simulink model "MPC_Design_1"  (R2023b)
settings: Solver=ode5  StartTime=0.0  StopTime=7  FixedStep=Ts  RelTol=1e-3
InitFcn:
  | Init_Model;
StartFcn:
  | Init_Model;
values from neighbouring files (symbols this model uses):
  ref = [0, 0]    [MPC_Design.m]
undefined symbols (not defined in the file or in its folder): Norm
libraries: slident x1, mpclib x1
settings Model: Creator=Selim  LastModifiedBy=Selim

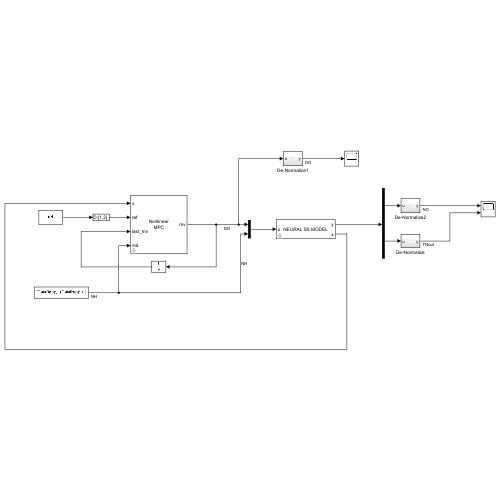
[thumbnail: Simulink's stored preview of the top-level diagram]
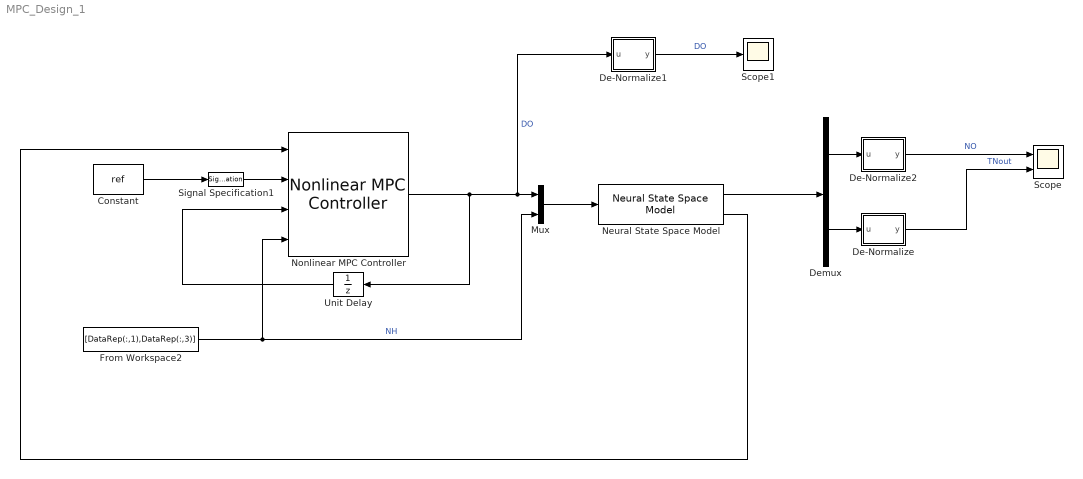
== system MPC_Design_1 ==
  Constant : Constant  Value=ref
  De-Normalize : Subsystem
  De-Normalize1 : Subsystem
  De-Normalize2 : Subsystem
  Demux : Demux  Outputs=2
  From Workspace2 : FromWorkspace  VariableName=[DataRep(:,1),DataRep(:,3)]
  Mux : Mux  Inputs=2
  Neural State Space Model : slident/Models/Neural State Space Model  sys=sys  x0type=internal  ic=x0  returnx=on  returndx=off  domain=CT  feedthroughCT=NoFT  feedthroughDT=FT
  Nonlinear MPC Controller : mpclib/Nonlinear MPC Controller  nlmpcobj=nlobj  UseObjectTs=on  UseMEX=off  md_enabled=on  mvtarget_enabled=off  param_enabled=off  cost_enabled=off  mvseq_enabled=off  stateseq_enabled=off  ovseq_enabled=off  slack_enabled=off  status_enabled=off  ov_min=off  ov_max=off  mv_min=off  mv_max=off  mvrate_min=off  mvrate_max=off  state_min=off  state_max=off  ov_weight=off  mv_weight=off  mvrate_weight=off  ecr_weight=off  nlp_initialize=off
  Scope : Scope  NumInputPorts=2
  Scope1 : Scope
  Signal Specification1 : SignalSpecification  Dimensions=[1,2]
  Unit Delay : UnitDelay  SampleTime=-1  HasFrameUpgradeWarning=on
  wires:
  Nonlinear MPC Controller/1 -> Unit Delay/1, De-Normalize1/1(u), Mux/1  "DO"
  Unit Delay/1 -> Nonlinear MPC Controller/3
  Mux/1 -> Neural State Space Model/1
  From Workspace2/1 -> Nonlinear MPC Controller/4, Mux/2  "NH"
  Demux/1 -> De-Normalize2/1(u)
  Demux/2 -> De-Normalize/1(u)
  De-Normalize2/1(y) -> Scope/1  "NO"
  De-Normalize/1(y) -> Scope/2  "TNout"
  Neural State Space Model/1 -> Demux/1
  Constant/1 -> Signal Specification1/1
  Neural State Space Model/2 -> Nonlinear MPC Controller/1
  De-Normalize1/1(y) -> Scope1/1  "DO"
  Signal Specification1/1 -> Nonlinear MPC Controller/2

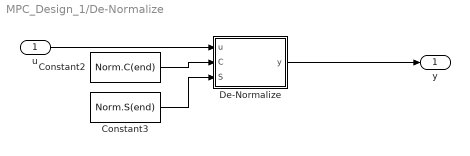
== system MPC_Design_1/De-Normalize ==
  u : Inport
  Constant2 : Constant  Value=Norm.C(end)
  Constant3 : Constant  Value=Norm.S(end)
  De-Normalize : MATLAB Function  TreatAsAtomicUnit=on
  y : Outport
  wires:
  Constant2/1 -> De-Normalize/2(C)
  De-Normalize/1(y) -> y/1
  u/1 -> De-Normalize/1(u)
  Constant3/1 -> De-Normalize/3(S)

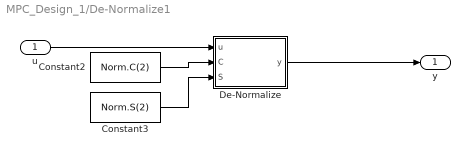
== system MPC_Design_1/De-Normalize1 ==
  u : Inport
  Constant2 : Constant  Value=Norm.C(2)
  Constant3 : Constant  Value=Norm.S(2)
  De-Normalize : MATLAB Function  TreatAsAtomicUnit=on
  y : Outport
  wires:
  Constant2/1 -> De-Normalize/2(C)
  De-Normalize/1(y) -> y/1
  u/1 -> De-Normalize/1(u)
  Constant3/1 -> De-Normalize/3(S)

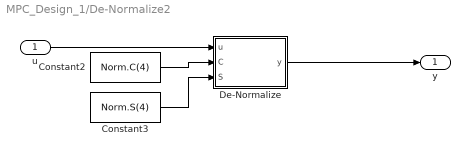
== system MPC_Design_1/De-Normalize2 ==
  u : Inport
  Constant2 : Constant  Value=Norm.C(4)
  Constant3 : Constant  Value=Norm.S(4)
  De-Normalize : MATLAB Function  TreatAsAtomicUnit=on
  y : Outport
  wires:
  Constant3/1 -> De-Normalize/3(S)
  u/1 -> De-Normalize/1(u)
  De-Normalize/1(y) -> y/1
  Constant2/1 -> De-Normalize/2(C)

== matlab function MPC_Design_1/De-Normalize1/De-Normalize ==
  data: u input; y output; C input; S input
function y = fcn(u,C,S)

y = u * S + C;

end

== matlab function MPC_Design_1/De-Normalize/De-Normalize ==
  data: u input; y output; C input; S input
function y = fcn(u,C,S)

y = u * S + C;

end

== matlab function MPC_Design_1/De-Normalize2/De-Normalize ==
  data: u input; y output; C input; S input
function y = fcn(u,C,S)

y = u * S + C;

end
